simulink model "control"  (R2019a)
settings: Solver=FixedStepAuto  StartTime=0.0  StopTime=0.5  FixedStep=0.001  RelTol=1e-3
values from neighbouring files (symbols this model uses):
  Gain = 27*6/(4095-2400)    (= 0.0955752212389)    [control.m]
  K = 2000*(z-0.7165)*(z-0.9)/(z*(z-1))    [control.m]
  Ref = 30    [control.m]
  tao = 0.01    [control.m]
libraries: simulink x2
settings Model: Creator=Maglemo  LastModifiedBy=Maglemo

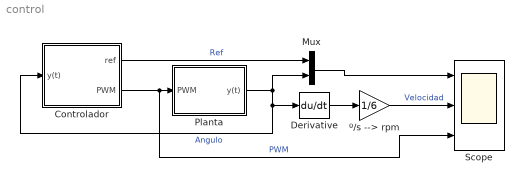
== system control ==
  Controlador : Subsystem
  Derivative : Derivative
  Mux : Mux  Inputs=2
  Planta : Subsystem
  Scope : Scope  NumInputPorts=3
  º/s --> rpm : Gain  Gain=1/6
  wires:
  Planta/1(y(t)) -> Mux/2, Controlador/1(y(t)), Derivative/1  "Angulo"
  Controlador/2(PWM) -> Scope/3, Planta/1(PWM)  "PWM"
  Controlador/1(ref) -> Mux/1  "Ref"
  Mux/1 -> Scope/1
  Derivative/1 -> º/s --> rpm/1
  º/s --> rpm/1 -> Scope/2  "Velocidad"

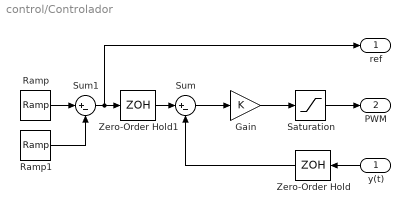
== system control/Controlador ==
  y(t) : Inport
  Gain : Gain  Gain=K
  Ramp : simulink/Sources/Ramp  slope=Ref/0.3  start=0.1  InitialOutput=0
  Ramp1 : simulink/Sources/Ramp  slope=Ref/0.3  start=0.1+0.3  InitialOutput=0
  Saturation : Saturate  UpperLimit=4095-2400  LowerLimit=0
  Sum : Sum  Inputs=|+-
  Sum1 : Sum  Inputs=|+-
  Zero-Order Hold : ZeroOrderHold  SampleTime=-1
  Zero-Order Hold1 : ZeroOrderHold  SampleTime=-1
  ref : Outport
  PWM : Outport  Port=2
  wires:
  Sum1/1 -> Zero-Order Hold1/1, ref/1
  Sum/1 -> Gain/1
  Saturation/1 -> PWM/1
  Zero-Order Hold/1 -> Sum/2
  Gain/1 -> Saturation/1
  y(t)/1 -> Zero-Order Hold/1
  Ramp/1 -> Sum1/1
  Ramp1/1 -> Sum1/2
  Zero-Order Hold1/1 -> Sum/1

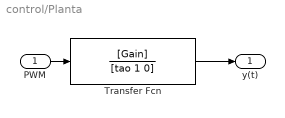
== system control/Planta ==
  PWM : Inport
  Transfer Fcn : TransferFcn  Numerator=[Gain]  Denominator=[tao 1 0]
  y(t) : Outport
  wires:
  Transfer Fcn/1 -> y(t)/1
  PWM/1 -> Transfer Fcn/1
